simulink model "PassiveCellBalancing"  (R2023b)
settings: Solver=FixedStepAuto  StartTime=0.0  StopTime=20  FixedStep=0.001  RelTol=1e-3
libraries: BatteryBalancing x1
settings Model: Creator=OWNER  LastModifiedBy=OWNER

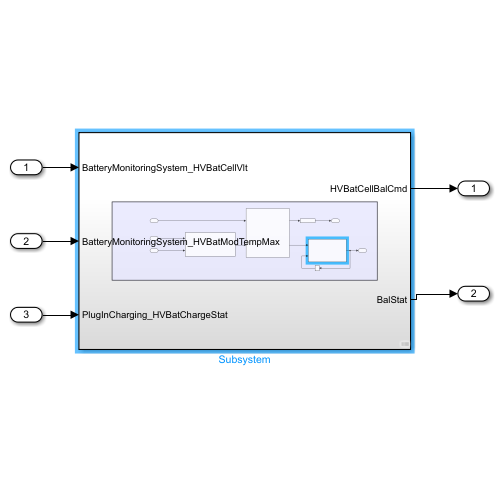
[thumbnail: Simulink's stored preview of the top-level diagram]
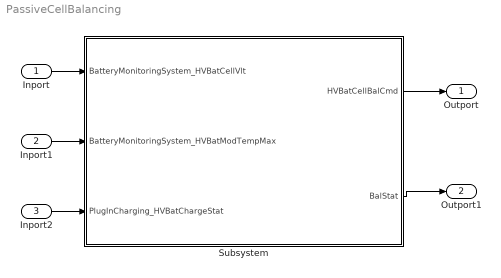
== system PassiveCellBalancing ==
  Inport : Inport
  Inport1 : Inport  Port=2
  Inport2 : Inport  Port=3
  Subsystem : Subsystem
  Outport : Outport
  Outport1 : Outport  Port=2
  wires:
  Inport/1 -> Subsystem/1(BatteryMonitoringSystem_HVBatCellVlt)
  Subsystem/1(HVBatCellBalCmd) -> Outport/1
  Inport1/1 -> Subsystem/2(BatteryMonitoringSystem_HVBatModTempMax)
  Inport2/1 -> Subsystem/3(PlugInCharging_HVBatChargeStat)
  Subsystem/2(BalStat) -> Outport1/1

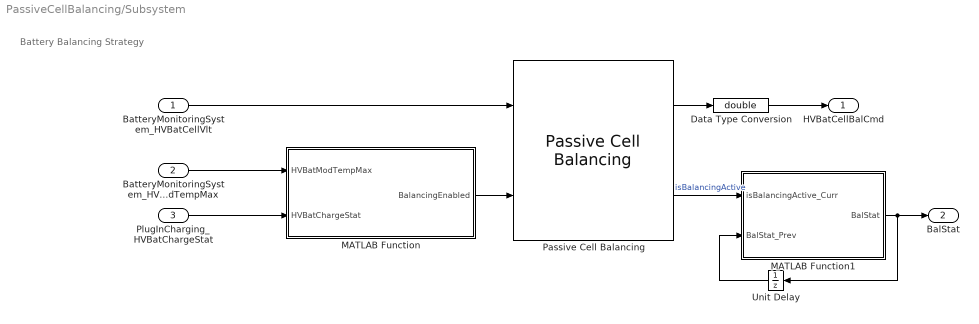
== system PassiveCellBalancing/Subsystem ==
  note: Battery Balancing Strategy
  BatteryMonitoringSystem_HVBatCellVlt : Inport
  BatteryMonitoringSystem_HVBatModTempMax : Inport  Port=2
  PlugInCharging_HVBatChargeStat : Inport  Port=3
  Data Type Conversion : DataTypeConversion  OutDataTypeStr=double  SaturateOnIntegerOverflow=off  RndMeth=Floor
  MATLAB Function : MATLAB Function  TreatAsAtomicUnit=on
  MATLAB Function1 : MATLAB Function  TreatAsAtomicUnit=on
  Passive Cell Balancing : BatteryBalancing/Passive Cell Balancing  Threshold=0.01  HysteresisBand=0  Td_on=10  Td_off=60  Ts=-1  dataType=double
      settings: LibrarySourceBlock=batt_sl_lib/Cell Balancing/Passive Cell Balancing
  Unit Delay : UnitDelay  SampleTime=-1  HasFrameUpgradeWarning=on
  HVBatCellBalCmd : Outport
  BalStat : Outport  Port=2
  wires:
  BatteryMonitoringSystem_HVBatCellVlt/1 -> Passive Cell Balancing/1
  Passive Cell Balancing/1 -> Data Type Conversion/1
  Passive Cell Balancing/2 -> MATLAB Function1/1(isBalancingActive_Curr)  "isBalancingActive"
  MATLAB Function/1(BalancingEnabled) -> Passive Cell Balancing/2
  Data Type Conversion/1 -> HVBatCellBalCmd/1
  MATLAB Function1/1(BalStat) -> BalStat/1, Unit Delay/1
  Unit Delay/1 -> MATLAB Function1/2(BalStat_Prev)
  BatteryMonitoringSystem_HVBatModTempMax/1 -> MATLAB Function/1(HVBatModTempMax)
  PlugInCharging_HVBatChargeStat/1 -> MATLAB Function/2(HVBatChargeStat)

== matlab function PassiveCellBalancing/Subsystem/MATLAB Function1 ==
  data: isBalancingActive_Curr input; BalStat output; BalStat_Prev input
function BalStat = balancingStatus(isBalancingActive_Curr, BalStat_Prev)

% Default: hold previous state
BalStat = BalStat_Prev;

if isBalancingActive_Curr == 1
    % Balancing currently active
    BalStat = 1;

elseif isBalancingActive_Curr == 0
    if BalStat_Prev == 1
        % Transition from active → inactive
        BalStat = 2;   % Completed
    elseif BalStat_Prev == 0 || BalStat_Prev == 2
        % Remain inactive or completed
        BalStat = BalStat_Prev;
    end
end

end

== matlab function PassiveCellBalancing/Subsystem/MATLAB Function ==
  data: HVBatModTempMax input; BalancingEnabled output; HVBatChargeStat input
function BalancingEnabled = balancingEnabled(HVBatModTempMax, HVBatChargeStat)
if HVBatModTempMax < 65 && HVBatChargeStat == 2
    BalancingEnabled = 1;
else
    BalancingEnabled = 0;
end
